simulink model "MySimplifiedTestingModel_20x2810x29"  (R2023a)
settings: Solver=ode1  StartTime=0.0  StopTime=inf  FixedStep=0.001  RelTol=1e-3
PostLoadFcn:
  | , if any(exist('dsrtsu_mdlpostloadfcn', 'file') ~= 0), dsrtsu_mdlpostloadfcn('Execute', bdroot); end,
InitFcn:
  | , if any(exist('rtifpga_mdlclblib', 'file') ~= 0), rtifpga_mdlclblib('Init', bdroot); end,
undefined symbols (not defined in the file or in its folder): START, STOP
libraries: rti1202serlib x11, simulink x6
(part 3 of 3)

== stateflow chart MySimplifiedTestingModel_20x2810x29/RS485/BUS MASTER FSM ==
  state INIT
    entry:
    TX_Trigger = false;
    TX_Len = 0;
    grant_ZKDM = false;
    grant_THERMO = false;
    resp_ok_ZKDM = false;
    resp_ok_THERMO = false;
    err_ZKDM = uint8(0);
    err_THERMO = uint8(0);
    currentDev = DEV_NONE;
    retry = 0;
    pollCounter = 0;
    rxCount = 0;
  state IDLE
    entry:
    currentDev = DEV_NONE;
    resp_ok_ZKDM=false;
    resp_ok_THERMO=false;
    resp_err_ZKDM=0;
    resp_err_THERMO=0;
    err_ZKDM=0;
    err_THERMO=0;
    grant_ZKDM=false;
    grant_THERMO=false;
    TX_Trigger=false;
    TX_Len=0;
    rxCount=0;
    during:
    if req_valid_ZKDM
    currentDev = DEV_ZKDM;
    elseif (pollCounter >= pollThermoEvery-1) && req_valid_THERMO
    currentDev = DEV_THERMO;
    pollCounter = 0;
    elseif req_valid_THERMO && ~req_valid_ZKDM
    currentDev = DEV_THERMO;
    else
    currentDev = DEV_NONE;
    end
  state VALIDATE1
    (junction 256) -> (junction 196) : {okAddr = addr_ok(rxBuf, rxCount, chosen_expect_addr);
        | okLen  = len_ok(rxCount, chosen_expect_len);
        | okCrc  = crc_ok(rxBuf, rxCount, chosen_expect_crc);}
    (junction 196) -> (junction 197) [order 1] : [~okAddr]
    (junction 196) -> (junction 198) [order 2]
    (junction 197) -> (junction 213)
    (junction 213) -> (junction 214) [order 1] : [currentDev==DEV_ZKDM]
    (junction 213) -> (junction 215) [order 2] : {err_THERMO = ERR_BAD_ADDR;}
    (junction 214) -> (junction 216) : {err_ZKDM = ERR_BAD_ADDR;}
    (junction 216) -> (junction 215)
    (junction 215) -> (junction 205)
    (junction 198) -> (junction 199) [order 1] : [~okLen]
    (junction 198) -> (junction 200) [order 2]
    (junction 199) -> (junction 220)
    (junction 220) -> (junction 221) [order 1] : [currentDev==DEV_ZKDM]
    (junction 220) -> (junction 223) [order 2] : {err_THERMO = ERR_BAD_LEN;}
    (junction 221) -> (junction 227) : {err_ZKDM = ERR_BAD_LEN;}
    (junction 227) -> (junction 223)
    (junction 223) -> (junction 204)
    (junction 200) -> (junction 201) [order 1] : [~okCrc]
    (junction 200) -> (junction 247) [order 2] : {resp_data = rxBuf;
        |     resp_len = rxCount;}
    (junction 201) -> (junction 231)
    (junction 231) -> (junction 232) [order 1] : [currentDev==DEV_ZKDM]
    (junction 231) -> (junction 234) [order 2] : {err_THERMO = ERR_BAD_CRC;}
    (junction 232) -> (junction 238) : {err_ZKDM = ERR_BAD_CRC;}
    (junction 247) -> (junction 248) [order 1] : [currentDev==DEV_ZKDM]
    (junction 238) -> (junction 234)
    (junction 247) -> (junction 249) [order 2] : {resp_ok_THERMO = true;}
    (junction 248) -> (junction 250) : {resp_ok_ZKDM = true;}
    (junction 234) -> (junction 235)
    (junction 250) -> (junction 249)
    (junction 249) -> (junction 202)
    (junction 235) -> (junction 202) [order 2]
    (junction 204) -> (junction 235)
    (junction 205) -> (junction 204)
  state LOAD_REQ
    entry:
    %chosen_req=0;
    %chosen_len=0;
    if currentDev == DEV_ZKDM
    chosen_req = req_bytes_ZKDM;
    chosen_len    = req_len_ZKDM;
    chosen_expect_addr = expect_addr_ZKDM;
    chosen_expect_len  = expect_len_ZKDM;
    chosen_expect_crc  = expect_crc_kind_ZKDM;
    timeout_ms = timeout_ms_ZKDM;
    grant_ZKDM = true;
    grant_THERMO = false;
    elseif currentDev == DEV_THERMO
    chosen_req = req_bytes_THERMO;
    chosen_len = req_len_THERMO;
    chosen_expect_addr = expect_addr_THERMO;
    chosen_expect_len  = expect_len_THERMO;
    chosen_expect_crc  = expect_crc_kind_THERMO;
    timeout_ms = timeout_ms_THERMO;
    grant_ZKDM = false;
    grant_THERMO = true;
    end
    TX_Data = chosen_req;
    TX_Len = chosen_len;
    retry = 0; rxCount = 0;
  state BACKOFF
    entry:
    % prepare next cycle selection
    if currentDev==DEV_ZKDM
    % advance thermostat poll counter
    pollCounter = min(pollCounter+1, pollThermoEvery-1);
    end
  state WAIT_THRE
  state TX_PULSE
    entry:
    TX_Trigger = true;
  state WAIT_RX_SWITCH
  state DELIVER_OK_CLEAR
    entry:
    resp_ok_ZKDM = false;
    resp_ok_THERMO = false;
  state DELIVER_OK_PULSE
  state TX_CLEAR
    entry:
    TX_Trigger = false;
  state WAIT_RX [commented out]
    during:
    % append latest chunk
    if RX_Len > 0
    if (rxCount + RX_Len) <= length(rxBuf)
    rxBuf(rxCount+1 : rxCount+RX_Len) = RX_Data(1:RX_Len);
    rxCount = rxCount + RX_Len;
    else
    % overflow protection
    if currentDev==DEV_ZKDM
    err_ZKDM = ERR_OVERFLOW;
    else
    err_THERMO = ERR_OVERFLOW;
    end
    % consume and move on
    rxCount = 0;
    goto('BACKOFF');
    end
    end
  note: goes to VALIDATE
  state WAIT_RX2
    (junction 397) -> (junction 396) [order 1] : [[(rxCount + RX_Len) <= length(rxBuf)] && RX_Len > 0 ]
    WAIT_RX2 -> (junction 397) [order 1]
    (junction 396) -> (junction 398) : {rxBuf(rxCount+1 : rxCount+RX_Len) = RX_Data(1:RX_Len);
        | rxCount = rxCount + RX_Len;}
    (junction 397) -> WAIT_RX2 [order 4] : [RX_Len == 0]
    (junction 397) -> (junction 400) [order 2] : [(rxCount + RX_Len) > length(rxBuf)]
    (junction 398) -> WAIT_RX2
    (junction 400) -> (junction 409) [order 1] : [currentDev==DEV_ZKDM]
    (junction 400) -> (junction 406) [order 2] : {err_THERMO = ERR_OVERFLOW;}
    (junction 409) -> (junction 410) : {err_ZKDM = ERR_OVERFLOW;}
    (junction 410) -> (junction 406)
  state RETRY_OR_BACKOFF1
    RETRY_OR_BACKOFF1 -> (junction 271) : [(after(1,tick))]
        | {rxBuf = zeros(1, 64, 'uint8');
        | rxCount = 0;}
    (junction 271) -> (junction 272) [order 1] : [retry < maxRetry]
    (junction 271) -> (junction 273) [order 2]
    (junction 272) -> (junction 274) : {retry = retry + 1;}
    (junction 274) -> (junction 273) [order 2]
    (junction 273) -> (junction 275)
  state VALIDATE [commented out]
    entry:
    okAddr = addr_ok(rxBuf, rxCount, chosen_expect_addr);
    okLen  = len_ok(rxCount, chosen_expect_len);
    okCrc  = crc_ok(rxBuf, rxCount, chosen_expect_crc);
    if ~okAddr
    if currentDev==DEV_ZKDM
    err_ZKDM = ERR_BAD_ADDR;
    else
    err_THERMO = ERR_BAD_ADDR;
    end
    goto('RETRY_OR_BACKOFF');
    elseif ~okLen
    if currentDev==DEV_ZKDM
    err_ZKDM = ERR_BAD_LEN;
    else
    err_THERMO = ERR_BAD_LEN;
    end
    goto('RETRY_OR_BACKOFF');
    elseif ~okCrc
    if currentDev==DEV_ZKDM
    err_ZKDM = ERR_BAD_CRC;
    else
    err_THERMO = ERR_BAD_CRC;
    end
    goto('RETRY_OR_BACKOFF');
    else
    % success → deliver
    resp_data = rxBuf(1:rxCount);
    resp_len = rxCount;
    if currentDev==DEV_ZKDM
    resp_ok_ZKDM = true;
    else
    resp_ok_THERMO = true;
    end
    goto('DELIVER_OK_PULSE');
    end
  state DELIVER_ERROR
    entry:
    if currentDev==DEV_ZKDM
    resp_err_ZKDM = err_ZKDM;
    else
    resp_err_THERMO = err_THERMO;
    end
  note: goes to RETRY_OR_BACKOFF1
  note: goes to DELIVER_ERR
  state DELIVER_ERR
    entry:
    if currentDev==DEV_ZKDM
    err_ZKDM = ERR_TIMEOUT;
    else
    err_THERMO = ERR_TIMEOUT;
    end
  state RETRY_OR_BACKOFF [commented out]
    entry:
    if retry < maxRetry
    retry = retry + 1;
    % Re-transmit same chosen_req
    goto('WAIT_THRE');
    else
    % give up and move on
    goto('BACKOFF');
    end
  state WAIT_RX1 [commented out]
    (junction 318) -> (junction 144) [commented out] : [(rxCount + RX_Len) <= length(rxBuf)]
    (junction 148) -> (junction 318) [commented out] : [RX_Len > 0]
    (junction 148) -> (junction 327) [commented out] : [after(timeout_ms, msec)]
    (junction 144) -> (junction 139) [commented out] : {rxBuf(rxCount+1 : rxCount+RX_Len) = RX_Data(1:RX_Len);
        |  rxCount = rxCount + RX_Len;}
    (junction 318) -> (junction 141) [commented out]
    (junction 141) -> (junction 142) [commented out] : [currentDev==DEV_ZKDM]
    (junction 141) -> (junction 138) [commented out] : {err_THERMO = ERR_OVERFLOW;}
    (junction 142) -> (junction 143) [commented out] : {err_ZKDM = ERR_OVERFLOW;}
    (junction 143) -> (junction 138) [commented out]
    (junction 138) -> (junction 319) [commented out] : {rxCount = 0;}
    (junction 319) -> (junction 327) [commented out]
    (junction 139) -> (junction 319) [commented out]
  (default) -> INIT
  INIT -> IDLE : [(after(1,tick))]
  BACKOFF -> IDLE : [after(interGap_ms, msec)]
  IDLE -> IDLE [commented out] : [currentDev==DEV_NONE]
  (junction 397) -> (junction 256) [order 3] : [rxCount >= chosen_expect_len]
  IDLE -> LOAD_REQ [order 1] : [currentDev==DEV_ZKDM]
  IDLE -> LOAD_REQ [order 2] : [currentDev==DEV_THERMO]
  LOAD_REQ -> WAIT_THRE : [(after(1,tick))]
  DELIVER_ERROR -> BACKOFF
  DELIVER_OK_CLEAR -> BACKOFF
  (junction 274) -> WAIT_THRE [order 1]
  WAIT_THRE -> TX_PULSE [order 1] : [THRE==true && tx_switch]
  WAIT_RX_SWITCH -> WAIT_THRE [order 1] : [tx_switch]
  WAIT_THRE -> WAIT_RX_SWITCH [order 2] : [~tx_switch]
  (junction 235) -> RETRY_OR_BACKOFF1 [order 1]
  (junction 202) -> DELIVER_OK_PULSE
  TX_PULSE -> TX_CLEAR : [(after(1,tick))]
  WAIT_RX_SWITCH -> WAIT_RX2 [order 2] : [rx_switch]
  DELIVER_OK_PULSE -> DELIVER_OK_CLEAR : [(after(1,tick))]
  TX_CLEAR -> WAIT_RX2
  (junction 275) -> DELIVER_ERROR
  DELIVER_ERR -> RETRY_OR_BACKOFF1
  (junction 406) -> RETRY_OR_BACKOFF1
  WAIT_RX2 -> DELIVER_ERR [order 1] : [after(timeout_ms, msec)]
  data: buf function_input; count function_input; expect_addr function_input; ok function_output; count function_input; expect_len function_input; ok function_output; buf function_input; count function_input; expected_crc function_input; ok function_output; THRE input boolean size=1; RX_Data input uint8 size=[1 64]; RX_Len input uint8 size=1; req_valid_ZKDM input boolean size=1; req_valid_THERMO input boolean size=1; now input size=1; TX_Data output uint8 size=[1 64]; TX_Len output uint8 size=1; TX_Trigger output boolean size=1; grant_ZKDM output boolean size=1; resp_err_ZKDM output uint8 size=1; resp_ok_ZKDM output boolean size=1; resp_data output uint8 size=[1 64]; resp_err_THERMO output uint8 size=1; resp_len output uint8 size=1; grant_THERMO output boolean size=1; resp_ok_THERMO output boolean size=1; expect_addr_THERMO input uint8 size=1; expect_addr_ZKDM input uint8 size=1; expect_crc_kind_THERMO input uint8 size=1; expect_crc_kind_ZKDM input uint8 size=1; tx_switch input boolean size=1; rx_switch input boolean size=1; expect_len_THERMO input uint8 size=1; expect_len_ZKDM input uint8 size=1; req_bytes_THERMO input uint8 size=[1 64]; req_bytes_ZKDM input uint8 size=[1 64]; req_len_THERMO input uint8 size=1; req_len_ZKDM input uint8 size=1; interGap_ms local uint16 =5; maxRetry local uint8 =1; pollThermoEvery local uint8 =4; timeout_ms_THERMO local uint16 =80; timeout_ms_ZKDM local uint16 =20; chosen_expect_addr local uint8; chosen_expect_crc local uint8 size=1; chosen_expect_len local uint8 size=1; chosen_len local uint8 size=1; chosen_req local uint8 size=[1 64]; currentDev local uint8 size=1 =0; okAddr local boolean size=1; okCrc local boolean size=1; okLen local boolean size=1; pollCounter local uint8 size=1 =0; retry local uint8 size=1 =0; rxBuf local uint8 size=[1 64]; rxCount local uint8 size=1 =0; timeout_ms local uint16 size=1 =20; DEV_NONE constant uint8 =0; DEV_THERMO constant uint8 =2; DEV_ZKDM constant uint8 =1; ERR_BAD_ADDR constant uint8 =2; ERR_BAD_CRC constant uint8 =4; ERR_BAD_LEN constant uint8 =3; ERR_OVERFLOW constant uint8 =5; ERR_TIMEOUT constant uint8 =1; err_THERMO local uint8 size=1; err_ZKDM local uint8 size=1
  function ok = addr_ok(buf, count, expect_addr):
    | function ok = addr_ok(buf, count, expect_addr)
    |     if count < 3
    |         ok = false;
    |     else
    |         ok = (buf(3) == expect_addr);
    |     end
    | end
  function ok = len_ok(count, expect_len):
    | function ok = len_ok(count, expect_len)
    |     ok = (count == expect_len);
    | end
  function ok = crc_ok(buf, count, expected_crc):
    | function ok = crc_ok(buf, count, expected_crc)
    |     % kind: 0=BCC XOR, 1=CRC16-RTU (LSB first)
    |      bcc = uint8(0);
    |     for k=1:(count-1)
    |         bcc = bitxor(bcc, buf(k));
    |     end
    |     ok = (buf(count) == bcc);
    | end

== stateflow chart MySimplifiedTestingModel_20x2810x29/RS485/Need to test the Status commands ==
  state Start [commented out]
    en: Access = false;
  state StartCmd
    en: prev1 = Start_Stop;
    en: prev2 = Temperature_value
    en: Access = true;
    en:
    if Start_Stop == true
    [RS485_Kommando, Kommando_NumBytes] = Command_Thermostat(0, 1);
    else
    [RS485_Kommando, Kommando_NumBytes] = Command_Thermostat(0, 0);
    end
    en:
    if after(2,sec)
    [RS485_Kommando, Kommando_NumBytes] = Command_Thermostat(1, double(Temperature_value));
    end
    exit: RS485_Kommando = zeros(1, 63);
    exit: Kommando_NumBytes = 0;
    exit: RS485_Kommando = zeros(1, 63);
    exit: Kommando_NumBytes = 0;
  state one
    en: initial = true;
  state box_650153605 %? [group]
    state Start1
      en: prev12 = Start_Stop2;
      en: prev22 =0;
      en: acc2 = true;
      en:
      if Start_Stop2 == true
      RS485_Kommando = FC_Command_8Bytes(false, true, ZKDM_value);
      else
      RS485_Kommando = FC_Command_8Bytes(false, false, ZKDM_value)
      end
    state Value
      en: prev22 = ZKDM_value;
      en: acc2 = true;
      en: RS485_Kommando = FC_Command_8Bytes(true, true,ZKDM_value);
    state Wait
      en: acc2 = false;
      en: RS485_Kommando = zeros(1, 63);
      en: NumBytes = 0;
    box_650153605.Start1 -> box_650153605.Wait : [after(2,sec)]
    box_650153605.Value -> box_650153605.Wait : [after(2,sec)]
    box_650153605.Wait -> box_650153605.Start1 [order 1] : [Start_Stop2 ~= prev12]
    box_650153605.Wait -> box_650153605.Value [order 2] : [(Start_Stop2 == true && ZKDM_value ~= prev22)]
  state box_570531625 %? [group]
    state Start1
      en: prev1 = Start_Stop;
      en: prev2 = 0;
      en: accthermo = true;
      en:
      if Start_Stop == true
      [RS485_Kommando, Kommando_NumBytes] = Command_Thermostat(0, 1);
      else
      [RS485_Kommando, Kommando_NumBytes] = Command_Thermostat(0, 0);
      end
    state Value
      en: prev2 = Temperature_value;
      en: accthermo = true;
      en: [RS485_Kommando, Kommando_NumBytes] = Command_Thermostat(1, double(Temperature_value));
    state Wait
      en: accthermo = false;
      en: RS485_Kommando = zeros(1, 63);
      en: NumBytes = 0;
    box_570531625.Start1 -> box_570531625.Wait : [after(2,sec)]
    box_570531625.Value -> box_570531625.Wait : [after(2,sec)]
    box_570531625.Wait -> box_570531625.Value [order 1] : [(Start_Stop ==true &&Temperature_value ~= prev2)]
    box_570531625.Wait -> box_570531625.Start1 [order 2] : [(Start_Stop ~= prev1)]
  state box_224206180 %? [group]
    state Badtemperature
      en:[RS485_Kommando, Kommando_NumBytes] = Command_Thermostat(2, NaN);
      en: accthermo = true;
      exit: Numbytes = 9;
      exit: overallReceived = zeros(1,63);
      exit: overallReceivedBytes = 0;
    state Waiting
      en: NumBytes = 0;
      en: overallReceived(uint8(overallReceivedBytes+1) : uint8(overallReceivedBytes+RXBytes)) = RXVector(1 : uint8(RXBytes));
      en: overallReceivedBytes = overallReceivedBytes + RXBytes;
    state Heizleistung
      en:[RS485_Kommando, Kommando_NumBytes] = Command_Thermostat(3, NaN);
      en: accthermo = true;
      exit: Numbytes = 9;
      exit: overallReceived = zeros(1,63);
      exit: overallReceivedBytes = 0;
    state Output1
      entry: ThermostatBadtemperatur = overallReceived;
      entry: accthermo = false;
    state Output2
      entry: ThermostatHeizleistung = overallReceived;
      en: accthermo = false;
    Badtemperature -> box_224206180.Waiting : [after(2,sec) && RXBytes>=9]
    Heizleistung -> box_224206180.Waiting : [after(2,sec) && RXBytes>=9]
    box_224206180.Waiting -> Output2 [order 2] : [overallReceived(overallReceivedBytes) == uint8(13)]
    box_224206180.Waiting -> Output1 [order 1] : [overallReceived(overallReceivedBytes) == uint8(13)]
    Output1 -> Heizleistung : [after(1,tick)]
  state box_48244028 %? [group]
    state AbfrageZKDM
      en: RS485_Kommando = FC_Command_8Bytes(true, true, ZKDM_value);
      en: NumBytes = 8;
      en: acc2 = true;
    state Waiting
      en: ZKDMZustand = RXVector;
      en: NumBytes = 0;
      en: acc2 = false;
    AbfrageZKDM -> box_48244028.Waiting : [after(2,sec) && RXBytes>=8]
  (default) -> one
  one -> Badtemperature [order 2] : [select == 2]
  one -> AbfrageZKDM [order 1] : [select == 3]
  one -> box_570531625.Start1 [order 4] : [select == 1]
  one -> box_650153605.Start1 [order 3] : [select == 0]
  box_48244028.Waiting -> box_570531625.Start1 [order 1] : [select == 0]
  box_650153605.Wait -> box_570531625.Start1 [order 4] : [select == 1]
  Output2 -> box_570531625.Start1 [order 2] : [select == 0]
  box_570531625.Wait -> box_650153605.Start1 [order 4] : [select == 0]
  Output2 -> box_650153605.Start1 [order 1] : [select == 1]
  box_48244028.Waiting -> box_650153605.Start1 [order 2] : [select == 1]
  box_570531625.Wait -> Badtemperature [order 5] : [select == 2]
  box_570531625.Wait -> AbfrageZKDM [order 3] : [select == 3]
  box_650153605.Wait -> AbfrageZKDM [order 5] : [select == 3]
  box_650153605.Wait -> Badtemperature [order 3] : [select == 2]
  data: RS485_Kommando output size=[1, 63]; NumBytes output uint32; Start_Stop input; Temperature_value input; prev1 local; prev2 local; prev12 local; prev22 local; ZKDM_value input; select input; Start_Stop2 input; initial local; overallReceived local uint8 size=[1 63]; overallReceivedBytes local size=[1 63]; ThermostatBadtemperatur output size=[1 63]; ThermostatHeizleistung output size=[1 63]; RXBytes input; RXVector input; Kommando_NumBytes local; ZKDMZustand output size=[63]; accthermo output; acc2 output

== matlab function MySimplifiedTestingModel_20x2810x29/RS485/Subsystem1/MATLAB Function ==
  data: u input; PCD1_1 output; PCD1_2 output; PCD2 output
function [PCD1_1, PCD1_2, PCD2] = fcn(u)
%Steuerwort
PCD1_1 = u(4);
PCD1_2 = u(5);

%berechnet aktuelle Ausgangsfrequenz als relativen Wert in Prozent
PCD2 = (u(6)*256 + u(7)) * (100 / 16384);

== matlab function MySimplifiedTestingModel_20x2810x29/RS485/MATLAB Function ==
  data: u input; y output

function y = fcn(u)
    y = '';

    % Find the index of the carriage return (byte 13)
    break_index = find(u == 13, 1);

    % If a carriage return is found, process up to that point
    if ~isempty(break_index)
        % Use only the bytes up to the first carriage return
        relevant_bytes = u(1:break_index - 1);
    else
        % If no carriage return is found, process the entire input
        relevant_bytes = u;
    end

    % Convert the relevant bytes to a string
    response_str = char(relevant_bytes);

    % Validate the response is not empty
    if isempty(response_str)
        % Return an empty string if the input is invalid
        return;
    end
    
    % Split the response based on underscore
    parts = strsplit(response_str, '_'); 

    % Validate the received data structure
    if length(parts) < 2
        % Return an empty string if the input structure is invalid
        return;
    end
    
    % Extract value from the received data
    y = parts{2};  % Second part is the value
end

== matlab function MySimplifiedTestingModel_20x2810x29/RS485/MATLAB Function1 ==
  data: u input; y output

function y = fcn(u)
    % Assumes maximum of 100 characters; adjust according to application
    coder.varsize('y', [1, 63], [0 1]);

    % Initialize the value of y
    y = uint8(zeros(1, 63));  % Use a uint8 array to represent the string in ASCII

    % Find the index of the carriage return (byte 13)
    break_index = find(u == 13, 1);

    % If a carriage return is found, process up to that point
    if ~isempty(break_index)
        % Use only the bytes up to the first carriage return
        relevant_bytes = u(1:break_index - 1);
    else
        % If no carriage return is found, process the entire input
        relevant_bytes = u;
    end

    % Convert the relevant bytes to a string
    response_str = char(relevant_bytes);

    % Validate the response is not empty
    if isempty(response_str)
        return;
    end
    
    % Split the response based on underscore
    parts = strsplit(response_str, '_'); 

    % Validate the received data structure
    if length(parts) < 2
        return;
    end
    
    % Extract value from the received data
    extracted_value = parts{2};  % Second part is the value

    % Convert the extracted value to uint8 for output
    y(1:numel(extracted_value)) = uint8(extracted_value);
end

== stateflow chart MySimplifiedTestingModel_20x2810x29/RS485/ZKDM FSM ==
  state INIT1 [commented out]
    % ZKDM replies are FC profile, fixed 8 bytes with BCC (XOR)
    expect_addr_ZKDM      = fc_addr;      % uint8 (the on-wire address byte you use)
    expect_len_ZKDM       = uint8(8);
    expect_crc_kind_ZKDM  = uint8(0);     % 0 = BCC/XOR
    % Device state defaults
    FU_bereit   = false;             % boolean
    freq_rel    = 0.0;               % double (0..100)
    status_word = uint16(0);         % uint16
    last_ok_ms  = uint32(0);         % optional freshness
    comm_err_count = uint16(0);      % uint16 counter
    % Request interface defaults
    req_valid   = false;
    req_len     = uint8(0);
    entry:
    req_valid = false;
    expect_addr_ZKDM = fc_addr;
    expect_len_ZKDM  = uint8(8);
    expect_crc_kind_ZKDM = uint8(0); % BCC XOR for FC
    FU_bereit = false;
    freq_rel = 0.0;
    status_word = uint16(0);
    last_ok_ms = uint32(0);
    comm_err_count = uint16(0);
  state INIT
    % ZKDM replies are FC profile, fixed 8 bytes with BCC (XOR)
    expect_addr_ZKDM      = fc_addr;      % uint8 (the on-wire address byte you use)
    expect_len_ZKDM       = uint8(8);
    expect_crc_kind_ZKDM  = uint8(0);     % 0 = BCC/XOR
    % parser outputs (safe defaults)
    PCD1_1 = uint8(0);
    PCD1_2 = uint8(0);
    status_word = uint16(0);
    freq_rel    = 0.0;
    fu_ctrl_ready    = false;
    fu_ready         = false;
    fault_trip       = false;
    fault_no_trip    = false;
    bus_ctrl_active = false;
    bcc_ok           = false;
    % Request interface defaults
    req_valid   = false;
    req_len     = uint8(0);
    %device
    last_ok_ms = uint32(0);
    comm_err_count = uint16(0);
  state READY
    entry:
    req_valid= false;
    READY_to_WAIT_GRANT = false;
    during:
    % Pacing: only build/send if enough time passed since last OK or last try
    if after(min_period_ms, msec)
    % Build the telegram NOW from live inputs
    tx_buf = fcn(invalid_flag, active, setpoint);
    % Advertise request to BUS MASTER
    req_bytes = tx_buf;
    req_len = tx_len;
    expect_addr_ZKDM  = tx_buf(3);
    expect_len_ZKDM   = uint8(8);
    expect_crc_kind_ZKDM = tx_buf(8); % BCC XOR
    req_valid    = true;
    % move to wait for arbitration
    READY_to_WAIT_GRANT = true;
    end
  state HANDLE_ERR
    entry:
    comm_err_count = comm_err_count + 1;
    % Optionally: set FU_bereit=false when repeated timeouts
  state COOLDOWN
    %nothing; the 'after(min_period_ms,msec)' in READY controls rate
  state PARSE
    entry:
    [PCD1_1, PCD1_2, freq_rel, status_word, ...
    fu_ctrl_ready, fu_ready, fault_trip, fault_no_trip, bus_ctrl_active, ...
    bcc_ok] = parse_fc_reply(resp_data);
    % Master should have validated addr/len/BCC already; still allow a local guard:
    if (bcc_ok)
    %tic();
    %last_ok_ms = uint32(toc());  % or leave; master’s timing is enough
    else
    comm_err_count = comm_err_count + uint16(1);
    end
  state WAIT_RESP
    during:
    % keep req_valid_ZKDM = false to avoid re-queuing while current tx is active
    req_valid = false;
  state WAIT_GRANT
    %hold req_valid_ZKDM high until master grants
    entry:
    READY_to_WAIT_GRANT = false;
  (default) -> INIT
  COOLDOWN -> READY : [after(1,tick)]
  INIT -> READY : [(after(1,tick))]
  HANDLE_ERR -> COOLDOWN : [(after(1,tick))]
  PARSE -> COOLDOWN : after(min_period_ms,msec)
  WAIT_RESP -> HANDLE_ERR [order 2] : [resp_err>0]
  WAIT_GRANT -> HANDLE_ERR [order 2] : [resp_err>0]
  READY -> WAIT_GRANT : [    READY_to_WAIT_GRANT == true]
  WAIT_RESP -> PARSE [order 1] : [resp_ok==true]
  WAIT_GRANT -> WAIT_RESP [order 1] : [grant==true]
  data: ctl_invalid function_input; run_en function_input; ref_pct function_input; bytes function_output; n function_output; q14 function_input; pct function_output; cfg function_output; buf function_input; n function_input; cfg function_input; ok function_output; status_word function_output uint16 size=1; freq_percent function_output; invalid_control_word function_input; active function_input; setpoint function_input; command function_output; u function_input uint8 size=[1 64]; PCD1_1 function_output uint8 size=1; PCD1_2 function_output uint8 size=1; freq_rel_percent function_output double size=1; status_word function_output uint16 size=1; fu_ctrl_ready function_output boolean size=1; fu_ready function_output boolean size=1; fault_trip function_output boolean size=1; fault_no_trip function_output boolean size=1; bus_control_active function_output boolean size=1; bcc_ok function_output boolean size=1; active input boolean size=1; setpoint input uint8 size=1; req_valid output boolean size=1; req_bytes output uint8 size=[1 64]; req_len output uint8 size=1; grant input boolean size=1; resp_ok input boolean size=1; resp_err input uint8 size=1; resp_data input uint8 size=[1 64]; resp_len input uint8 size=1; fc_addr local uint8 size=1 =253; invalid_flag input boolean size=1; min_period_ms local uint8 size=1 =50; FU_bereit local boolean size=1; expect_addr_ZKDM output uint8 size=1; expect_crc_kind_ZKDM output uint8 size=1; expect_len_ZKDM output uint8 size=1; freq_rel local double size=1; last_ok_ms local uint32 size=1; READY_to_WAIT_GRANT local boolean size=1; cfg local uint8 size=1; f_percent local uint8 size=1; ok local boolean size=1; status_word local uint16 size=1; sw local uint16 size=1; tx_buf local uint8 size=[1 64]; tx_len local uint8 size=1 =8; PCD1_1 local uint8 size=1; PCD1_2 local uint8 size=1; bcc_ok local boolean size=1; bus_control_active local boolean size=1; fault_no_trip local boolean size=1; fault_trip local boolean size=1; fu_ctrl_ready local boolean size=1; fu_ready local boolean size=1; comm_err_count local uint16 size=1; bus_ctrl_active local boolean size=1; tx_trigger input boolean size=1
  function [bytes, n] = build_pcd8(ctl_invalid, run_en, ref_pct):
    | function [bytes, n] = build_pcd8(ctl_invalid, run_en, ref_pct)
    |     % Call your tested MATLAB Function (Create FC-Protocol Command 8-Bytes)
    |     % Or inline the builder. Must return [1x8 uint8] and n=8.
    |     n = unit8(8);
    |     [bytes, n] = FC_Command_8Bytes(ctl_invalid, run_en, ref_pct);
    | end
  function pct = q14_to_percent(q14):
    | function pct = q14_to_percent(q14)
    |     pct = 100.0 * double(q14) / 16384.0;
    | end
  function cfg = zkdm_resp_map:
    | function cfg = zkdm_resp_map()
    | % Positions are 1-based indices in the received byte vector
    | cfg.idx_stx   = 1;
    | cfg.idx_len   = 2;
    | cfg.idx_addr  = 3;
    | cfg.idx_statH = 4;
    | cfg.idx_statL = 5;
    | cfg.idx_freqH = 6;
    | cfg.idx_freqL = 7;
    | cfg.idx_bcc   = 8;
    | 
    | cfg.expect_len = 8;        % total bytes
    | cfg.endian_hi_lo = true;   % Q14 is [HI, LO]
    | cfg.q14_fullscale = 16384; % 100%
    | end
  function [ok, status_word, freq_percent] = parse_fc_status(buf, n, cfg):
    | function [ok, status_word, freq_percent] = parse_fc_status(buf, n, cfg)
    | % buf: uint8 vector of the validated reply
    | % n  : actual length (== cfg.expect_len if master validated length)
    | % cfg: map from zkdm_resp_map()
    | 
    | ok = false;
    | status_word = uint16(0);
    | freq_percent = 0.0;
    | 
    | % Basic shape check (defensive)
    | if n < cfg.expect_len
    |     return;
    | end
    | 
    | % Status word (Bytes 4..5 by default)
    | stat_hi = uint16(buf(cfg.idx_statH));
    | stat_lo = uint16(buf(cfg.idx_statL));
    | status_word = bitor( stat_lo, bitshift(stat_hi, 8) );  % (HI,LO) → 16-bit
    | 
    | % Q14 output frequency (Bytes 6..7 by default)
    | bH = uint16(buf(cfg.idx_freqH));
    | bL = uint16(buf(cfg.idx_freqL));
    | if cfg.endian_hi_lo
    |     q14 = bitor( bL, bitshift(bH, 8) );     % HI,LO on the wire → H<<8 | L
    | else
    |     q14 = bitor( bH, bitshift(bL, 8) );     % LO,HI variant if needed
    | end
    | 
    | % Clip and scale to percent
    | if q14 > cfg.q14_fullscale
    |     q14 = cfg.q14_fullscale;   % sanity
    | end
    | freq_percent = 100.0 * double(q14) / double(cfg.q14_fullscale);
    | 
    | ok = true;
    | end
  function command = fcn(invalid_control_word, active, setpoint):
    | % Generates a telegram of the FC protocol for communication with a Danfoss frequency converter,
    | % telegram type: Process block (PCD) – 4 bytes
    | %
    | %##################################################################################
    | %Danfoss control word according to FC profile
    | %----------------------------------------------------------------------------------
    | %| Bit|                        Bit value = 0 |                     Bit value = 1  |
    | %|----|--------------------------------------|------------------------------------|
    | %| 00 | selection between the four "3-10 Preset reference [0]...[3]"             |
    | %| 01 | --""--                                                                   |
    | %|----|--------------------------------------|------------------------------------|
    | %| 02 |             DC brake and stop        |             performs ramp          |
    | %|----|--------------------------------------|------------------------------------|
    | %| 03 | lets the motor coast                 | starts the motor if conditions are met |
    | %|----|--------------------------------------|------------------------------------|
    | %| 04 | motor speed decreases until stop     |                                    |
    | %|----|--------------------------------------|------------------------------------|
    | %| 05 | current output frequency is stored   |                                    |
    | %|----|--------------------------------------|------------------------------------|
    | %| 06 | stop using ramp time                 | starts the motor if conditions are met |
    | %|----|--------------------------------------|------------------------------------|
    | %| 07 | no reset                             | reset                              |
    | %|----|--------------------------------------|------------------------------------|
    | %| 08 |                                      | output frequency "3-19 Jog [RPM]"  |
    | %|----|--------------------------------------|------------------------------------|
    | %| 09 | ramp 1 active ("3-41" and "3-42")    | ramp 2 active ("3-51" and "3-52")  |
    | %|----|--------------------------------------|------------------------------------|
    | %| 10 | control word is ignored              | control word is used               |
    | %|----|--------------------------------------|------------------------------------|
    | %| 11 | relay 01 not activated               | relay 01 activated                 |
    | %|----|--------------------------------------|------------------------------------|
    | %| 12 | relay 04 not activated               | relay 04 activated                 |
    | %|----|--------------------------------------|------------------------------------|
    | %| 13 | parameter set selection "0-10" and "8-55"                                |
    | %| 14 |                                                                            |
    | %|----|--------------------------------------|------------------------------------|
    | %| 15 | no reversal                          | reversal                           |
    | %----------------------------------------------------------------------------------
    | %##################################################################################
    | 
    | function command = fcn(invalid_control_word, active, setpoint)
    | 
    | if setpoint < 0
    |         error('setpoint must be non-negative.');
    | end
    | 
    | command = zeros(1, 64, 'uint8');
    | startzeichen = uint8(2);    % Start character (STX)
    | telegrammlaenge = uint8(6); % Specifies telegram length: 6 or 14 data bytes (data bytes + address byte + checksum)
    | adresse = 0b01111101;       % Address 125 in binary, address of the frequency converter (FU)
    |                             % Address format 1–126 => Bit 7 = 1; FU address “10” => Bit 0–6
    | pcd1_1 = 0b00000000;        % Control word (CTW) bits 08 to 15
    | pcd1_2 = 0b00101110;        % Control word (CTW) bits 00 to 07
    | bcc = 0;                    % Data control byte, Block Check Character (BCC)
    | 
    | % modify the flag
    | if (invalid_control_word == false)
    |     pcd1_1 = bitor(pcd1_1, 0b00100000); 
    |     % If invalid_flag is `false`, the result will change `pcd11` to `0b00100000`, indicating that the control word is now in use.
    | end
    | 
    | if (active == true)
    |     pcd1_1 = bitor(pcd1_1, 0b00010000); % Starts the motor; “0”: the frequency converter lets the motor coast
    | end
    | 
    | %%- `command(4) = pcd1_1;`
    |   % - Value: This byte is constructed based on the input conditions (`steuerwort_invalid` and `aktiv`).
    |   % - It starts with `0b00000000` (initial value) and may have bits set:
    |   %   - Bit 5 is set to 1 if `steuerwort_invalid` is false (valid control word).
    |   %   - Bit 4 is set to 1 if `aktiv` is true (start command).
    |   % - As a result, if `aktiv` is true, the value changes:
    |   %     - From: `0b00100000`
    |   %     - To:   `0b00110000` (decimal 48), indicating that the motor should start.
    | 
    | % scale the speed setpoint
    | % Example: convert 50% speed to 16-bit integer
    | % 50% = (16384 / 100 * 50) = 8192
    | % 8192 = 0b1000000000000000 (binary)
    | 
    | soll = setpoint * (16384 / 100); 
    | pcd2 = typecast(int16(soll),'uint8');
    | pcd2 = flip(pcd2);
    | %This is a 16-bit integer converted to two bytes that represents the desired speed (drehzahl_Sollwert) scaled to a proper range.
    |    %- The speed is scaled by multiplying the `drehzahl_Sollwert` by `(16384 / 100)`, allowing for a representation of the speed setting as a 16-bit integer.
    |    %- This is then converted from an `int16` to `uint8`, giving two bytes: `pcd2(1)` and `pcd2(2)`, with the bytes being flipped to match byte order expectations.
    | 
    | bcc = bitxor(startzeichen, telegrammlaenge);
    | bcc = bitxor(bcc, adresse);
    | bcc = bitxor(bcc, pcd1_1);
    | bcc = bitxor(bcc, pcd1_2);
    | bcc = bitxor(bcc, pcd2(1));
    | bcc = bitxor(bcc, pcd2(2));
    | 
    | command(1) = startzeichen;
    | command(2) = telegrammlaenge;
    | command(3) = adresse;
    | command(4) = pcd1_1; %This byte functions as part of the control command to the motor, determining how it should behave.
    | command(5) = pcd1_2; %This byte also forms part of the control command. It usually contains predefined flags or control commands as per the motor's specification.
    | command(6:7) = pcd2; %This part of the command specifies the desired speed for the motor. from the user sollwert.
    | command(8) = bcc;
    | 
    | %example message:
    | 
    | %Address: 118 Motor Activation Flag: True Target Speed: 89% BCC is valid
    | %2 6 118 48 46 56 246 162
  function [PCD1_1, PCD1_2, freq_rel_percent, ...:
    | function [PCD1_1, PCD1_2, freq_rel_percent, ...
    |           status_word, ...
    |           fu_ctrl_ready, fu_ready, fault_trip, fault_no_trip, bus_control_active, ...
    |           bcc_ok] = parse_fc_reply(u)
    | %#codegen
    | % Parse 8-byte FC reply built by your current build_fc_rx_telegram()
    | % Layout: [STX, LEN, ADDR, STW_HI, STW_LO, OUT_HI, OUT_LO, BCC]
    | % Bit mapping (matches your TX builder with msbpos()):
    | %   fu_ctrl_ready      -> bit15
    | %   fu_ready           -> bit14
    | %   fault_trip         -> bit13
    | %   fault_no_trip      -> bit12
    | %   bus_control_active -> bit6
    | 
    |     % ---- basic checks ----
    |     if numel(u) < 8
    |         error('parse_fc_reply:BadLength','u must have at least 8 bytes');
    |     end
    |     u = uint8(u(:).'); % row uint8
    | 
    |     % ---- BCC (XOR of bytes 1..7) ----
    |     b = uint8(0);
    |     for k = 1:7
    |         b = bitxor(b, u(k));
    |     end
    |     bcc_ok = (b == u(8));
    | 
    |     % ---- status word bytes ----
    |     PCD1_1 = u(4); % high byte (bits 15..8)
    |     PCD1_2 = u(5); % low  byte (bits 7..0)
    | 
    |     % Full 16-bit status word: [HI<<8 | LO]
    |     status_word = bitor( bitshift(uint16(PCD1_1),8), uint16(PCD1_2) );
    | 
    |     % Helper to read a single LSB-indexed bit (0..15)
    |     getbit = @(w, n) bitand(w, bitshift(uint16(1), n)) ~= 0;
    | 
    |     % ---- flags (LSB indexing) matching your TX mapping ----
    |     fu_ctrl_ready      = getbit(status_word, 15); % msbpos(0)
    |     fu_ready           = getbit(status_word, 14); % msbpos(1)
    |     fault_trip         = getbit(status_word, 13); % msbpos(2)
    |     fault_no_trip      = getbit(status_word, 12); % msbpos(3)
    |     bus_control_active = getbit(status_word,  6); % msbpos(9)
    | 
    |     % ---- OUT (Q14) -> relative frequency (%) ----
    |     q14 = bitor( bitshift(uint16(u(6)),8), uint16(u(7)) );
    |     freq_rel_percent = double(q14) * (100.0/16384.0);
    | end

== stateflow chart MySimplifiedTestingModel_20x2810x29/RS485/Testing only Sending ON//OFF and Value commands ==
  state one
    en: initial = true;
  state THERMO [group]
    state Start1
      en: accthermo = true;
      en: prev2 = Temperature_value;
      en:
      if Start_Stop == true
      [RS485_Kommando, Kommando_NumBytes] = Command_Thermostat(0, 1);
      else
      [RS485_Kommando, Kommando_NumBytes] = Command_Thermostat(0, 0);
      end
    state Value
      en: prev2 = Temperature_value;
      en: accthermo = true;
      en: [RS485_Kommando, Kommando_NumBytes] = Command_Thermostat(1, double(Temperature_value));
    state Wait
      en: accthermo = false;
      en: prev1 = Start_Stop;
      en: RS485_Kommando = zeros(1, 63);
      en: NumBytes = 0;
    state gf
      en: prev2 = Temperature_value;
    THERMO.Start1 -> THERMO.Wait : [after(1,tick)]
    THERMO.Value -> THERMO.Wait : [after(1,tick)]
    THERMO.Wait -> THERMO.Value [order 2] : [(Start_Stop ==true && Temperature_value ~= prev2)]
    THERMO.Wait -> THERMO.Start1 [order 1] : [(Start_Stop ~= prev1)]
    gf -> THERMO.Wait
  state ZKDM [group]
    state Start1
      en: acc2 = true;
      en: prev22 = ZKDM_value;
      en:
      if Start_Stop2 == true
      RS485_Kommando = FC_Command_8Bytes(false, true, ZKDM_value);
      else
      RS485_Kommando = FC_Command_8Bytes(false, false, ZKDM_value)
      end
    state Value
      en: prev22 = ZKDM_value;
      en: acc2 = true;
      en: RS485_Kommando = FC_Command_8Bytes(true, true,ZKDM_value);
    state d
      en: prev22  = ZKDM_value;
    state Wait
      en: acc2 = false;
      en: prev12 = Start_Stop2;
      en: RS485_Kommando = zeros(1, 63);
      en: NumBytes = 0;
    ZKDM.Start1 -> ZKDM.Wait : [after(1,tick)]
    ZKDM.Value -> ZKDM.Wait : [after(1,tick)]
    ZKDM.Wait -> ZKDM.Value [order 2] : [(Start_Stop2 == true && ZKDM_value ~= prev22)]
    ZKDM.Wait -> ZKDM.Start1 [order 1] : [Start_Stop2 ~= prev12]
    d -> ZKDM.Wait : [after(1,tick)]
  (default) -> one
  one -> THERMO.Start1 [order 1] : [select == 0]
  one -> ZKDM.Start1 [order 2] : [select == 1]
  THERMO.Wait -> d [order 3] : [select ==1]
  ZKDM.Wait -> gf [order 3] : [select == 0]
  data: Kommando_NumBytes output; Start_Stop input; Start_Stop2 input; Temperature_value input; ZKDM_value input; select input; NumBytes output; RS485_Kommando output; acc2 output; accthermo output; initial output; prev1 local; prev12 local; prev2 local; prev22 local

== stateflow chart MySimplifiedTestingModel_20x2810x29/RS485/THERMO FSM ==
  data: active input; setpoint input; req_valid output; req_bytes output; req_len output; expect_addr output; grant input; resp_ok input; resp_err input; resp_data input; len input

== matlab function MySimplifiedTestingModel_20x2810x29/RS485/Create FC-Protocol Command 8-Bytes/Create 8-Bytes Command1 ==
  data: steuerwort_invalid input; aktiv input; command output; drehzahl_Sollwert input
function command = fcn(steuerwort_invalid, aktiv, drehzahl_Sollwert)
    if drehzahl_Sollwert < 0
        error('drehzahl_Sollwert must be non-negative.');
    end
    command = zeros(1, 8, 'uint8'); % Corrected the size from 63 to 8 for simplicity

    startzeichen = uint8(2);    % Startzeichen (STX)
    telegrammlaenge = uint8(6); % Angabe der Telegrammlaenge
    adresse = 0b10001010;       % Adresse 138 in binary
    pcd1_1 = 0b00000000;        % Steuerwort (CTW) Bit 08 bis 15
    pcd1_2 = 0b00101110;        % Steuerwort (CTW) Bit 00 bis 07
    bcc = 0;                    % Block Check Character (BCC)

    % Modify the control word
    if (steuerwort_invalid == false)
        pcd1_1 = bitor(pcd1_1, 0b00100000);
    end

    if (aktiv == true)
        pcd1_1 = bitor(pcd1_1, 0b00010000);
    end

    % Scale the speed setpoint
    soll = drehzahl_Sollwert * (16384 / 100);
    pcd2 = typecast(int16(soll), 'uint8');
    pcd2 = flip(pcd2);

    % Calculate the Block Check Character
    bcc = bitxor(startzeichen, telegrammlaenge);
    bcc = bitxor(bcc, adresse);
    bcc = bitxor(bcc, pcd1_1);
    bcc = bitxor(bcc, pcd1_2);
    bcc = bitxor(bcc, pcd2(1));
    bcc = bitxor(bcc, pcd2(2));

    command(1) = startzeichen;
    command(2) = telegrammlaenge;
    command(3) = adresse;
    command(4) = pcd1_1;
    command(5) = pcd1_2;
    command(6:7) = pcd2;
    command(8) = bcc;
end

== matlab function MySimplifiedTestingModel_20x2810x29/RS485/MATLAB Function2 ==
  data: u input; PCD1_1 output; PCD1_2 output; freq_rel_percent output; status_word output; fu_ctrl_ready output; fu_ready output; fault_trip output; fault_no_trip output; bus_control_active output; bcc_ok output
function [PCD1_1, PCD1_2, freq_rel_percent, ...
          status_word, ...
          fu_ctrl_ready, fu_ready, fault_trip, fault_no_trip, bus_control_active, ...
          bcc_ok] = parse_fc_reply(u)
%#codegen
% Parse 8-byte FC reply built by your current build_fc_rx_telegram()
% Layout: [STX, LEN, ADDR, STW_HI, STW_LO, OUT_HI, OUT_LO, BCC]
% Bit mapping (matches your TX builder with msbpos()):
%   fu_ctrl_ready      -> bit15
%   fu_ready           -> bit14
%   fault_trip         -> bit13
%   fault_no_trip      -> bit12
%   bus_control_active -> bit6

    % ---- basic checks ----
    if numel(u) < 8
        error('parse_fc_reply:BadLength','u must have at least 8 bytes');
    end
    u = uint8(u(:).'); % row uint8

    % ---- BCC (XOR of bytes 1..7) ----
    b = uint8(0);
    for k = 1:7
        b = bitxor(b, u(k));
    end
    bcc_ok = (b == u(8));

    % ---- status word bytes ----
    PCD1_1 = u(4); % high byte (bits 15..8)
    PCD1_2 = u(5); % low  byte (bits 7..0)

    % Full 16-bit status word: [HI<<8 | LO]
    status_word = bitor( bitshift(uint16(PCD1_1),8), uint16(PCD1_2) );

    % Helper to read a single LSB-indexed bit (0..15)
    getbit = @(w, n) bitand(w, bitshift(uint16(1), n)) ~= 0;

    % ---- flags (LSB indexing) matching your TX mapping ----
    fu_ctrl_ready      = getbit(status_word, 15); % msbpos(0)
    fu_ready           = getbit(status_word, 14); % msbpos(1)
    fault_trip         = getbit(status_word, 13); % msbpos(2)
    fault_no_trip      = getbit(status_word, 12); % msbpos(3)
    bus_control_active = getbit(status_word,  6); % msbpos(9)

    % ---- OUT (Q14) -> relative frequency (%) ----
    q14 = bitor( bitshift(uint16(u(6)),8), uint16(u(7)) );
    freq_rel_percent = double(q14) * (100.0/16384.0);
end

== stateflow chart MySimplifiedTestingModel_20x2810x29/RS232/FSM2: zyklische Datenabfrage ==
  state Initialisierung
    entry: RS232_Kommando = zeros(1, 63);
    entry: NumBytes = 0;
    entry: Zugriff = false;
  state WarteAufFreigabe
    entry: FSM_Step = 1;
  state WartetEinePeriode
    entry: Zugriff = true;
    entry: FSM_Step = 2;
  state ZykluszeitUeberschritten
    entry: ZykluszeitUeberschritten = true;
    entry: Zugriff = false;
    entry: FSM_Step = 15;
  state WarteAufNeuenZyklus
    entry: ZykluszeitUeberschritten = false;
    entry: Zugriff = false;
    entry: FSM_Step = 14;
  state PrueftObFreigabNochGegeben
    entry: FSM_Step = 3;
  state AbfrageIstwert
    entry: NextCycleActionPoint = Clock + MaxCycleTime;
    entry: RS232_Kommando(1:7) = uint8('IN_PV_1');
    entry: RS232_Kommando(8) = uint8(13);
    entry: RS232_Kommando(9) = uint8(10);
    entry: Kommando_NumBytes = 9;
    entry: TriggerTX = true;
    entry: ResponseTimeoutPoint = Clock + MaxResponseTime;
    exit: RS232_Kommando = zeros(1, 63);
    exit: Kommando_NumBytes = 0;
    exit: TriggerTX = false;
    entry: FSM_Step = 4;
  state PrueftObFIFOLeer_2
    entry: FSM_Step = 13;
  state LeertFIFO_2
    entry: NumBytes = 1;
    entry: FSM_Step = 12;
  state Zeitueberschreitung
    entry: KeineAntwort = true;
    entry: Zugriff = false;
    entry: NumBytes = 0;
    entry: FSM_Step = 100;
  state WarteAufAntwortIstwert
    entry: NumBytes = 4;
    entry: FSM_Step = 5;
  state AktualisiertStatus
    entry: Statusmeldung = RXString;
    entry: NumBytes = 0;
    entry: FSM_Step = 11;
  state AktualisiertIstwert
    entry: Istwert = RXString;
    entry: KeineAntwort = false;
    entry: NumBytes = 0;
    entry: FSM_Step = 6;
  state WarteAufAntwortStatus
    entry: NumBytes = 1;
    entry: FSM_Step = 10;
  state LeertFIFO_1
    entry: NumBytes = 1;
    entry: FSM_Step = 7;
  state AbfrageStatus
    entry: RS232_Kommando(1:6) = uint8('STATUS');
    entry: RS232_Kommando(7) = uint8(13);
    entry: RS232_Kommando(8) = uint8(10);
    entry: Kommando_NumBytes = 8;
    entry: TriggerTX = true;
    entry: ResponseTimeoutPoint = Clock + MaxResponseTime;
    exit: RS232_Kommando = zeros(1, 63);
    exit: Kommando_NumBytes = 0;
    exit: TriggerTX = false;
    entry: FSM_Step = 9;
  state PrueftObFIFOLeer_1
    exit: NumBytes = 0;
    entry: FSM_Step = 8;
  (default) -> Initialisierung
  Initialisierung -> WarteAufFreigabe
  ZykluszeitUeberschritten -> WarteAufFreigabe : [after(1,tick)]
  WarteAufFreigabe -> WartetEinePeriode : [Freigegeben == true]
  WarteAufNeuenZyklus -> WarteAufFreigabe : [(Clock-NextCycleActionPoint) >= 0]
  Zeitueberschreitung -> WarteAufFreigabe : [after(1,tick)]
  PrueftObFreigabNochGegeben -> WarteAufFreigabe [order 1] : [Freigegeben == false]
  WartetEinePeriode -> PrueftObFreigabNochGegeben : [after(1,tick)]
  PrueftObFIFOLeer_2 -> ZykluszeitUeberschritten [order 2] : [(Clock-NextCycleActionPoint) >= 0]
  PrueftObFIFOLeer_2 -> WarteAufNeuenZyklus [order 3]
  PrueftObFreigabNochGegeben -> AbfrageIstwert [order 2] : [Freigegeben == true]
  PrueftObFIFOLeer_2 -> LeertFIFO_2 [order 1] : [NumRXBytes > 0]
  LeertFIFO_2 -> PrueftObFIFOLeer_2 : [after(1,tick)]
  AbfrageIstwert -> WarteAufAntwortIstwert : [after(1,tick)]
  AktualisiertStatus -> LeertFIFO_2 : [after(1,tick)]
  WarteAufAntwortIstwert -> Zeitueberschreitung [order 2] : [(Clock-ResponseTimeoutPoint) >= 0]
  WarteAufAntwortStatus -> Zeitueberschreitung [order 2] : [(Clock-ResponseTimeoutPoint) >= 0]
  WarteAufAntwortIstwert -> AktualisiertIstwert [order 1] : [NumRXBytes >= 4]
  WarteAufAntwortStatus -> AktualisiertStatus [order 1] : [NumRXBytes >= 1]
  AktualisiertIstwert -> LeertFIFO_1 : [after(1,tick)]
  AbfrageStatus -> WarteAufAntwortStatus : [after(1,tick)]
  PrueftObFIFOLeer_1 -> LeertFIFO_1 [order 1] : [NumRXBytes > 0]
  LeertFIFO_1 -> PrueftObFIFOLeer_1 : [after(1,tick)]
  PrueftObFIFOLeer_1 -> AbfrageStatus [order 2]
  data: RS232_Kommando output; Kommando_NumBytes output; TriggerTX output; Zugriff output; Istwert output; Statusmeldung output; RXString input; NumRXBytes input; Clock input; ResponseTimeoutPoint local; MaxResponseTime constant double =2; KeineAntwort output boolean =false; ZykluszeitUeberschritten output boolean =false; NumBytes output uint32; NextCycleActionPoint local; MaxCycleTime constant double =5; FSM_Step output; Freigegeben input
